simulink model "trial1x3"  (R2018b)
settings: Solver=VariableStepAuto  StartTime=0.0  StopTime=10.0  MaxStep=0.01  RelTol=1e-3
settings Model: Creator=Ismael  LastModifiedBy=Ismael

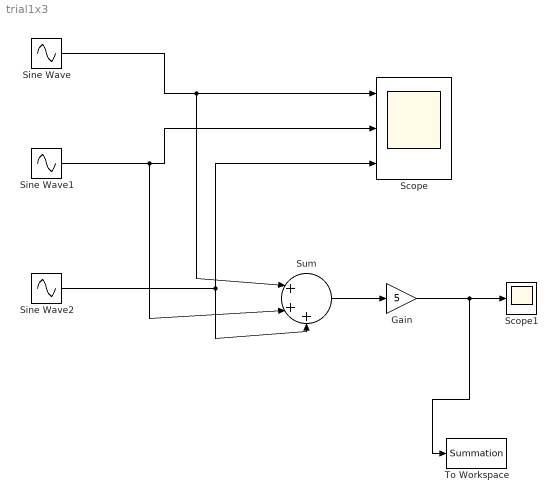
== system trial1x3 ==
  Gain : Gain  Gain=5
  Scope : Scope  NumInputPorts=3
  Scope1 : Scope
  Sine Wave : Sin  SampleTime=0
  Sine Wave1 : Sin  Frequency=5  SampleTime=0
  Sine Wave2 : Sin  Frequency=10  SampleTime=0
  Sum : Sum  Inputs=|+++
  To Workspace : ToWorkspace  VariableName=Summation  SaveFormat=Timeseries  SampleTime=-1
  wires:
  Sine Wave2/1 -> Sum/3, Scope/3
  Sine Wave/1 -> Sum/1, Scope/1
  Sine Wave1/1 -> Sum/2, Scope/2
  Sum/1 -> Gain/1
  Gain/1 -> To Workspace/1, Scope1/1
